simulink model "testDetect"  (R2023a)
settings: Solver=FixedStepDiscrete  StartTime=0.0  StopTime=10.0  FixedStep=0.040  RelTol=1e-3
values from neighbouring files (symbols this model uses):
  background = [62 62 62 62 62 62 62 62 62 62 62 62 ... (307200 elements, 480x640)]    [background.mat]    (also in slDetect.m = rgb2gray(imread('background.png')))
undefined symbols (not defined in the file or in its folder): imtest, Rec, SDTV, strel
libraries: visionstatistics x1, visionmorphops x1, visionconversions x1, visionsinks x1
settings Model: Creator=vmano  LastModifiedBy=vmano

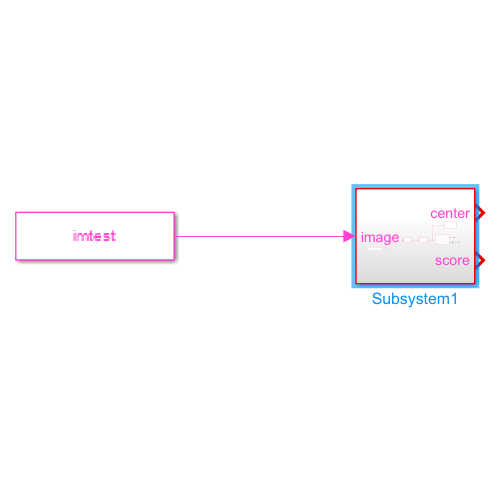
[thumbnail: Simulink's stored preview of the top-level diagram]
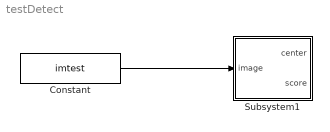
== system testDetect ==
  Constant : Constant  Value=imtest
  Subsystem1 : Subsystem
  wires:
  Constant/1 -> Subsystem1/1(image)

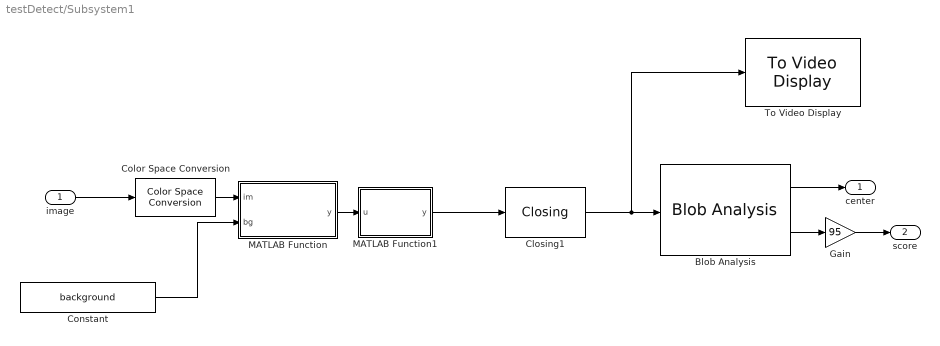
== system testDetect/Subsystem1 ==
  image : Inport
  Blob Analysis : visionstatistics/Blob Analysis  Tag=vipblks_row_conv  area=off  centroid=on  bBox=off  majorAxis=off  minorAxis=off  angle=off  eccentricity=off  equivDiameterSq=off  extent=off  perimeter=off  outDT=double  conn=8  isLabel=off  maxBlobs=1  warnIfNumBlobsExceeded=on  isCount=on  useMinArea=on  minArea=625  useMaxArea=off  maxArea=intmax('uint32')  excludeBorderBlob=off  isOutVarDim=off  isFill=on  fillValues=-1  roundingMode=Floor  overflowMode=off  prodOutputMode=Binary point scaling  prodOutputWordLength=32  prodOutputFracLength=16  accumMode=Binary point scaling  accumWordLength=32  accumFracLength=0  outputMode=Binary point scaling  outputWordLength=32  outputFracLength=16  firstCoeffMode=Binary point scaling  firstCoeffWordLength=16  firstCoeffFracLength=14  secondCoeffMode=Binary point scaling  secondCoeffWordLength=32  secondCoeffFracLength=16
  Closing1 : visionmorphops/Closing  nhoodsrc=Specify via dialog  strel=strel('disk',5)
  Color Space Conversion : visionconversions/Color Space  Conversion  conversion=Obsolete  conversionActive=R'G'B' to intensity  wp_str=D65  rec=Rec. 601 (SDTV)  sys=1125/60/2:1  imagePorts=One multidimensional signal
  Constant : Constant  Value=background
  Gain : Gain  Gain=95
  MATLAB Function : MATLAB Function  TreatAsAtomicUnit=on
  MATLAB Function1 : MATLAB Function  TreatAsAtomicUnit=on
  To Video Display : visionsinks/To Video Display  windowSizeMode=Normal  openAtMdlStart=on  fullScreen=off  videoWindowX=97  videoWindowY=60  saveWindowSize=off  videoWindowWidth=640  videoWindowHeight=480  inputColorFormat=RGB  inputType=Obsolete  imagePorts=One multidimensional signal  OutputDevice=On-screen video monitor  dataOrg=Column-major  isWindowOpen=off
  center : Outport
  score : Outport  Port=2
  wires:
  image/1 -> Color Space Conversion/1
  Constant/1 -> MATLAB Function/2(bg)
  MATLAB Function/1(y) -> MATLAB Function1/1(u)
  MATLAB Function1/1(y) -> Closing1/1
  Closing1/1 -> To Video Display/1, Blob Analysis/1
  Color Space Conversion/1 -> MATLAB Function/1(im)
  Gain/1 -> score/1
  Blob Analysis/2 -> Gain/1
  Blob Analysis/1 -> center/1

== matlab function testDetect/Subsystem1/MATLAB Function ==
  data: im input; y output; bg input
function y = bgRemove(im, bg)

im16 = int16(im);
bg16 = int16(bg);

y16 = im16-bg16;
y16(y16<0) = 0;

y = uint8(y16);

== matlab function testDetect/Subsystem1/MATLAB Function1 ==
  data: u input; y output
function y = threshold(u)

th = 50;

y8 = u;
y8(y8<th)= 0;
y8(y8>th)= 1;

y = logical(y8);
